simulink model "Test_Bit_Multiplexer_16_to_1"  (Simulink 8.1)
settings: Solver=ode45  StartTime=0.0  StopTime=len  RelTol=1e-3
libraries: commutil2 x2, Bit_Multiplexers_Lib x1
settings Model: Creator=N  LastModifiedBy=uzivatel
settings DataIOCC: LimitDataPoints=off  SignalLoggingSaveFormat=Dataset
settings OptimizationCC: ExpressionDepthLimit=128
settings DebuggingCC: UnderspecifiedInitializationDetection=Simplified  MergeDetectMultiDrivingBlocksExec=error  SolverPrmCheckMsg=none  FcnCallInpInsideContextMsg=EnableAllAsError  FrameProcessingCompatibilityMsg=error  StateNameClashWarn=none
settings HardwareCC: ProdBitPerPointer=64  ProdLargestAtomicFloat=Float  ProdIntDivRoundTo=Zero  ProdEndianess=LittleEndian  ProdHWDeviceType=Intel->x86-64 (Windows64)
settings ModelReferenceCC: PropagateSignalLabelsOutOfModel=on
settings GRTTargetCC: CodeReplacementLibrary=None  CombineOutputUpdateFcns=on  CPPClassGenCompliant=on  GRTInterface=off

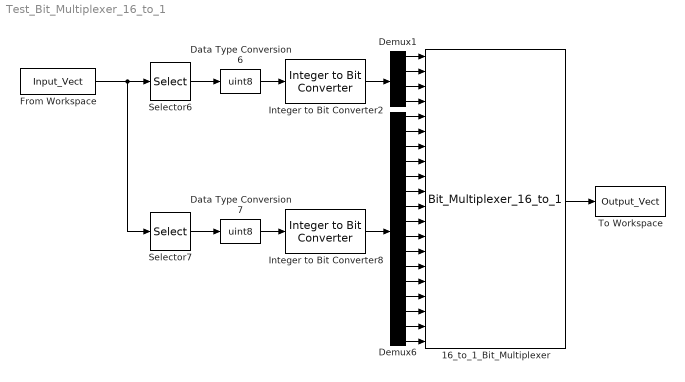
== system Test_Bit_Multiplexer_16_to_1 ==
  16_to_1_Bit_Multiplexer : Bit_Multiplexers_Lib/Bit_Multiplexers_Lib/Bit_Multiplexer_16_to_1
  Data Type Conversion6 : DataTypeConversion  OutDataTypeStr=uint8
  Data Type Conversion7 : DataTypeConversion  OutDataTypeStr=uint8
  Demux1 : Demux
  Demux6 : Demux  Outputs=16
  From Workspace : FromWorkspace  VariableName=Input_Vect  SampleTime=1  Interpolate=off  OutputAfterFinalValue=Holding final value
  Integer to Bit Converter2 : commutil2/Integer to Bit Converter  nbits=4  signedInputValues=Unsigned  bitOrder=MSB first  outDtype=boolean
  Integer to Bit Converter8 : commutil2/Integer to Bit Converter  nbits=16  signedInputValues=Unsigned  bitOrder=MSB first  outDtype=uint8
  Selector6 : Selector  IndexMode=Zero-based  InputPortWidth=2  SampleTime=1  IndexOptions=Index vector (dialog)  Indices=0  OutputSizes=1
  Selector7 : Selector  IndexMode=Zero-based  InputPortWidth=2  IndexOptions=Index vector (dialog)  Indices=1  OutputSizes=1
  To Workspace : ToWorkspace  VariableName=Output_Vect  SampleTime=1
  wires:
  Integer to Bit Converter8/1 -> Demux6/1
  Demux1/1 -> 16_to_1_Bit_Multiplexer/1
  Demux1/2 -> 16_to_1_Bit_Multiplexer/2
  Demux1/3 -> 16_to_1_Bit_Multiplexer/3
  Demux1/4 -> 16_to_1_Bit_Multiplexer/4
  Integer to Bit Converter2/1 -> Demux1/1
  Demux6/1 -> 16_to_1_Bit_Multiplexer/5
  Demux6/2 -> 16_to_1_Bit_Multiplexer/6
  Demux6/3 -> 16_to_1_Bit_Multiplexer/7
  Demux6/4 -> 16_to_1_Bit_Multiplexer/8
  Demux6/5 -> 16_to_1_Bit_Multiplexer/9
  Demux6/6 -> 16_to_1_Bit_Multiplexer/10
  Demux6/7 -> 16_to_1_Bit_Multiplexer/11
  Demux6/8 -> 16_to_1_Bit_Multiplexer/12
  Demux6/9 -> 16_to_1_Bit_Multiplexer/13
  Demux6/10 -> 16_to_1_Bit_Multiplexer/14
  Demux6/11 -> 16_to_1_Bit_Multiplexer/15
  Demux6/12 -> 16_to_1_Bit_Multiplexer/16
  Demux6/13 -> 16_to_1_Bit_Multiplexer/17
  Demux6/14 -> 16_to_1_Bit_Multiplexer/18
  Demux6/15 -> 16_to_1_Bit_Multiplexer/19
  Demux6/16 -> 16_to_1_Bit_Multiplexer/20
  From Workspace/1 -> Selector7/1, Selector6/1
  Selector6/1 -> Data Type Conversion6/1
  Selector7/1 -> Data Type Conversion7/1
  Data Type Conversion6/1 -> Integer to Bit Converter2/1
  Data Type Conversion7/1 -> Integer to Bit Converter8/1
  16_to_1_Bit_Multiplexer/1 -> To Workspace/1
